simulink subsystem "range_esstimation"  (R2023a)
settings: Solver=VariableStepAuto  StartTime=0.0  StopTime=10.0  RelTol=1e-3
values from neighbouring files (symbols this model uses):
  battery_high_cut_off = 95    [run_model.m]
  battery_low_cut_off = 5    [run_model.m]
  Capacity_kWh = Capacity_Ah*NominalVoltage/1000*(battery_high_cut_off-battery_low_cut_off)/100    (= 83.25)    [run_model.m]
libraries: simulink x1
settings Model: Creator=sandu  LastModifiedBy=sandu

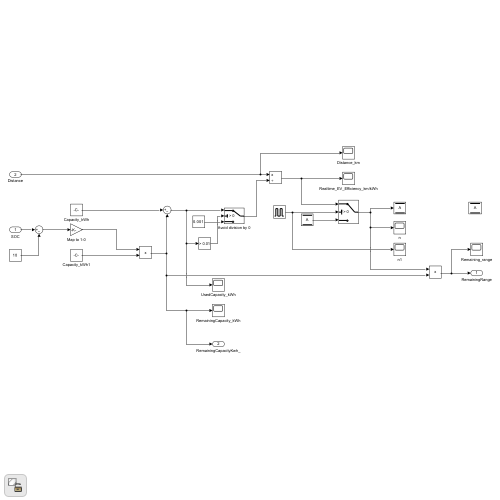
[thumbnail: Simulink's stored preview of the top-level diagram]
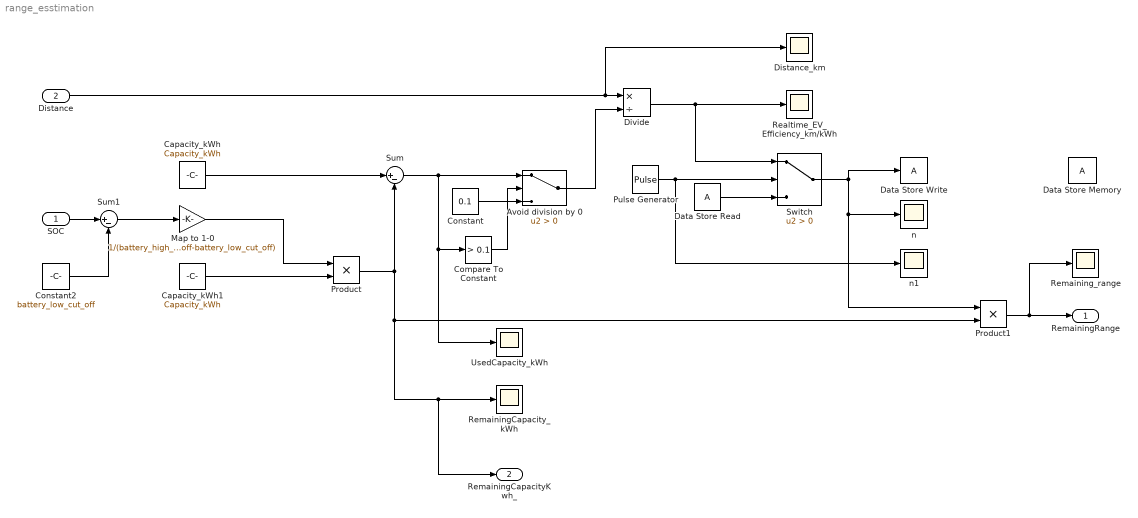
== system range_esstimation ==
  SOC : Inport
  Distance : Inport  Port=2
  Avoid division by 0 : Switch  Criteria=u2 > Threshold  SaturateOnIntegerOverflow=off  InputSameDT=off
  Capacity_kWh : Constant  Value=Capacity_kWh
  Capacity_kWh1 : Constant  Value=Capacity_kWh
  Compare To Constant : simulink/Logic and Bit Operations/Compare To Constant  relop=>  const=0.1  OutDataTypeStr=boolean
  Constant : Constant  Value=0.1
  Constant2 : Constant  Value=battery_low_cut_off
  Data Store Memory : DataStoreMemory  WriteAfterWriteMsg=warning  InitialValue=1.46  ShowAdditionalParam=off
  Data Store Read : DataStoreRead  IndexOptions=Index vector (dialog)  Indices=1  OutputSizes=1
  Data Store Write : DataStoreWrite  IndexOptions=Index vector (dialog)  Indices=1  OutputSizes=1
  Distance_km : Scope
  Divide : Product  Inputs=*/
  Map to 1-0 : Gain  Gain=1/(battery_high_cut_off-battery_low_cut_off)
  Product : Product
  Product1 : Product
  Pulse Generator : DiscretePulseGenerator  PulseType=Time based  Period=500  PhaseDelay=500
  Realtime_EV_Efficiency_km/kWh : Scope
  RemainingCapacity_kWh : Scope
  Remaining_range : Scope
  Sum : Sum  Inputs=|+-
  Sum1 : Sum  Inputs=|+-
  Switch : Switch  Criteria=u2 > Threshold  SaturateOnIntegerOverflow=off  InputSameDT=off
  UsedCapacity_kWh : Scope
  n : Scope
  n1 : Scope
  RemainingRange : Outport
  RemainingCapacityKwh_ : Outport  Port=2
  wires:
  Capacity_kWh1/1 -> Product/2
  Map to 1-0/1 -> Product/1
  Capacity_kWh/1 -> Sum/1
  Product/1 -> Product1/2, RemainingCapacity_kWh/1, RemainingCapacityKwh_/1, Sum/2
  Distance/1 -> Divide/1, Distance_km/1
  Sum/1 -> Avoid division by 0/1, Compare To Constant/1, UsedCapacity_kWh/1
  Avoid division by 0/1 -> Divide/2
  Compare To Constant/1 -> Avoid division by 0/2
  Constant/1 -> Avoid division by 0/3
  Product1/1 -> RemainingRange/1, Remaining_range/1
  SOC/1 -> Sum1/1
  Sum1/1 -> Map to 1-0/1
  Constant2/1 -> Sum1/2
  Divide/1 -> Realtime_EV_Efficiency_km/kWh/1, Switch/1
  Switch/1 -> n/1, Product1/1, Data Store Write/1
  Pulse Generator/1 -> Switch/2, n1/1
  Data Store Read/1 -> Switch/3
